simulink model "test_transform"  (R2018b)
settings: Solver=FixedStepAuto  StartTime=0  StopTime=5  FixedStep=Ts  RelTol=1e-3
values from neighbouring files (symbols this model uses):
  x_e = x_e_1    [AcDcInterlink.m]    (also in GridFollowingBuck.m; GridFormingBuck.m = [i_ld; i_lq; i_ld_i; i_lq_i; v_od; v_oq; v_od_i; v_oq_i; i_o)
undefined symbols (not defined in the file or in its folder): DeviceDiscreDamping, DevicePara, DevicePowerFlow, DeviceType, OtherInputs, PowerFlow, Sbase, Ts, Vbase, Wbase, Zbase
libraries: powerlib x11, SimplexPS x4
settings Model: Creator=yg934  LastModifiedBy=yg934

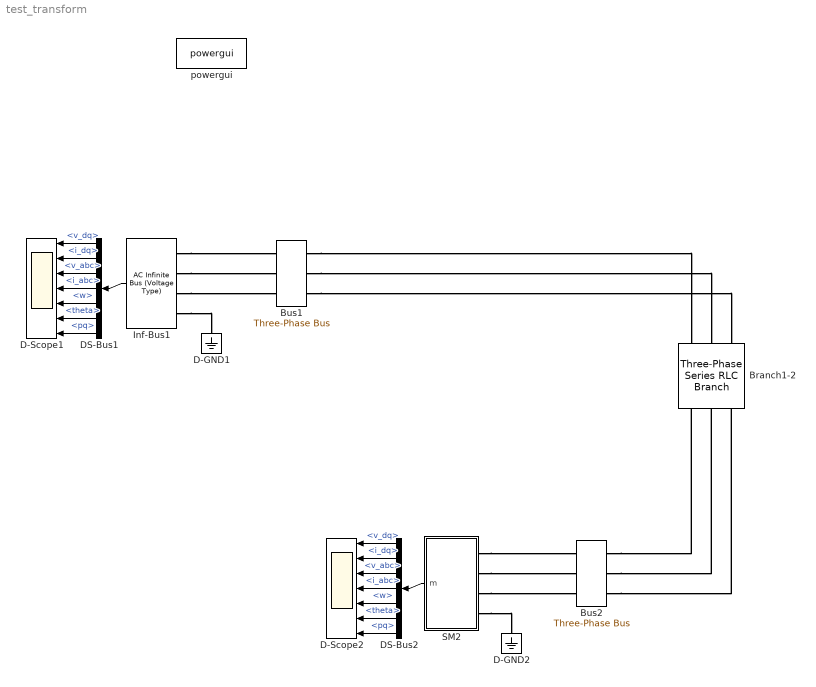
== system test_transform ==
  Branch1-2 : powerlib/Elements/Three-Phase Series RLC Branch  LConnTagsString=A|B|C  RConnTagsString=A|B|C  BranchType=L  Resistance=(0)*Zbase  Inductance=(0.65)*Zbase/Wbase  Capacitance=1e-6  Measurements=None
  Bus1 : SimplexPS/Three-Phase Bus  Vbase=1  Sbase=1
  Bus2 : SimplexPS/Three-Phase Bus  Vbase=1  Sbase=1
  D-GND1 : powerlib/Elements/Ground  LConnTagsString=a
  D-GND2 : powerlib/Elements/Ground  LConnTagsString=a
  D-Scope1 : Scope  NumInputPorts=7
  D-Scope2 : Scope  NumInputPorts=7
  DS-Bus1 : BusSelector  OutputSignals=v_dq,i_dq,v_abc,i_abc,w,theta,pq
  DS-Bus2 : BusSelector  OutputSignals=v_dq,i_dq,v_abc,i_abc,w,theta,pq
  Inf-Bus1 : SimplexPS/AC Infinite Bus (Voltage Type)  Ts=Ts  Sbase=Sbase  Vbase=Vbase  Wbase=Wbase  vd=PowerFlow{1}(3)  vq=0  theta0=PowerFlow{1}(4)  w=Wbase  R=1e-30
  SM2 : Subsystem  AncestorBlock=|  mask{Ts=Ts, Sbase=Sbase, Vbase=Vbase, Wbase=Wbase, DeviceType=DeviceType{2}, DevicePara=DevicePara{2}, PowerFlow=DevicePowerFlow{2}, x0=x_e{2}, OtherInputs=OtherInputs{2}, DiscreMethod=Hybrid Trapezoidal, EnableInsideModification=off, DiscreDampingFlag=on, DiscreDampingValue=DeviceDiscreDamping{2}, LinearizationTimes=1, DirectFeedthrough=off}
      | SimplexPS/Synchronous Machine
      | (dq-Frame System Object)
      mask prompts: Ts "Ts (s), samping period"; Sbase "Sbase (VA), power base"; Vbase "Vbase (V), voltage base"; Wbase "Wbase (rad/s), frequency base"; DeviceType "Device type"; DevicePara "Device parameters"; PowerFlow "Power flow paramters"; x0 "x0, initial states"; OtherInputs "Other inputs"; DiscreMethod "Discrerization method"; EnableInsideModification "Enable inside modification"; DiscreDampingFlag "Enable discretization damping"; DiscreDampingValue "Discretization damping value"; LinearizationTimes "Linearization times"; DirectFeedthrough "Direct feedthrough"
      mask init:
      | SimplexPS.Simulink.DeviceMaskInitialization(EnableInsideModification,DiscreDampingFlag);
      mask TypeOptions DiscreMethod: Forward Euler | Hybrid Trapezoidal | Virtual Damping
      mask TypeOptions LinearizationTimes: 1 | 2
  powergui : powerlib/powergui  Priority=1  SimulationMode=Discrete  SampleTime=Ts  frequency=60  Iterations=50  frequencyindice=0  Pbase=100e6  ErrMax=1e-4  UnitsV=kV  UnitsW=MW  buscounter=0  FunctionMessages=off  echomessages=off  EnableUseOfTLC=off  CurrentSourceSwitches=off  DisableSnubberDevices=off  DisableRonSwitches=off  DisableVfSwitches=off  DisplayEquations=off  SolverType=Tustin/Backward Euler (TBE)  Interpol=off  ExternalGateDelay=off  methode=off  Ts=100  x0status=blocks  SPID=off  SwTol=0  HookPort=off  RestoreLinks=warning  ResistiveCurrentMeasurement=off  Frange=[0:2:500]  Ylog=off  Xlog=on  ShowGrid=off  save=off  variable=ZData  structure=0  ZoomFFT=off  StartTime=0.0  cycles=1  DisplayStyle=1  fundamental=60  FreqAxis=off  MaxFrequency=1000  frequencyindicesteady=1  RmsSteady=1  display=off
  wires:
  Inf-Bus1/1 -> DS-Bus1/1
  DS-Bus1/1 -> D-Scope1/1  "<v_dq>"
  DS-Bus1/2 -> D-Scope1/2  "<i_dq>"
  DS-Bus1/3 -> D-Scope1/3  "<v_abc>"
  DS-Bus1/4 -> D-Scope1/4  "<i_abc>"
  DS-Bus1/5 -> D-Scope1/5  "<w>"
  DS-Bus1/6 -> D-Scope1/6  "<theta>"
  DS-Bus1/7 -> D-Scope1/7  "<pq>"
  SM2/1(m) -> DS-Bus2/1
  DS-Bus2/1 -> D-Scope2/1  "<v_dq>"
  DS-Bus2/2 -> D-Scope2/2  "<i_dq>"
  DS-Bus2/3 -> D-Scope2/3  "<v_abc>"
  DS-Bus2/4 -> D-Scope2/4  "<i_abc>"
  DS-Bus2/5 -> D-Scope2/5  "<w>"
  DS-Bus2/6 -> D-Scope2/6  "<theta>"
  DS-Bus2/7 -> D-Scope2/7  "<pq>"
  connections:
  Inf-Bus1/LConn4 -- D-GND1/LConn1
  SM2/LConn4 -- D-GND2/LConn1
  Bus2/RConn1 -- Branch1-2/RConn1
  Bus2/RConn2 -- Branch1-2/RConn2
  Bus2/RConn3 -- Branch1-2/RConn3
  Bus1/RConn1 -- Branch1-2/LConn1
  Bus1/RConn2 -- Branch1-2/LConn2
  Bus1/RConn3 -- Branch1-2/LConn3
  Inf-Bus1/LConn1 -- Bus1/LConn1
  Inf-Bus1/LConn2 -- Bus1/LConn2
  Inf-Bus1/LConn3 -- Bus1/LConn3
  SM2/LConn1 -- Bus2/LConn1
  SM2/LConn2 -- Bus2/LConn2
  SM2/LConn3 -- Bus2/LConn3

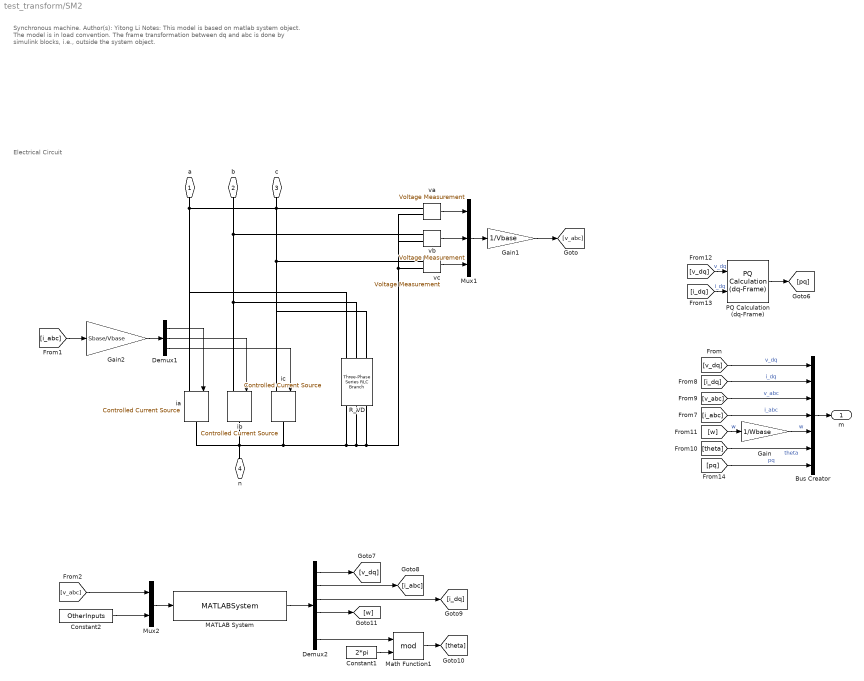
== system test_transform/SM2 ==
  note: Electrical Circuit
  note: Synchronous machine.
      |
      | Author(s): Yitong Li
      |
      | Notes:
      |
      | This model is based on matlab system object.
      |
      | The model is in load convention.
      |
      | The frame transformation between dq and abc is done by simulink blocks, i.e., outside the system object.
  Bus Creator : BusCreator  Inputs=7
  Constant1 : Constant  Value=2*pi
  Constant2 : Constant  Value=OtherInputs
  Demux1 : Demux  Outputs=3
  Demux2 : Demux  Outputs=[2,3,2,1,1,1]
  Gain : Gain  Gain=1/Wbase
  Gain1 : Gain  Gain=1/Vbase
  Gain2 : Gain  Gain=Sbase/Vbase
  MATLAB System : MATLABSystem  System=SimplexPS.Class.SynchronousMachineTransform  Ts=Ts  Para=DevicePara  DeviceType=DeviceType  PowerFlow=PowerFlow  x0=x0  DiscreMethod=DiscreMethod  LinearizationTimes=LinearizationTimes  DirectFeedthrough=DirectFeedthrough  VirtualResistor=DiscreDampingFlag  EquiInitial=true  ElecPortIOs=[ 1, 2 ]  SimulateUsing=Code generation
      mask Type: SimplexPS.Class.SynchronousMachineTransform
      mask Display:
      | disp('SynchronousMachineTransform');
      | port_label('input',1,'u');
      | port_label('output',1,'y');
  Math Function1 : Math  Operator=mod  SaturateOnIntegerOverflow=on
  Mux1 : Mux  Inputs=3
  Mux2 : Mux  Inputs=[3,2]
  PQ Calculation (dq-Frame) : SimplexPS/PQ Calculation (dq-Frame)  SystemSampleTime=-1
  R_VD : powerlib/Elements/Three-Phase Series RLC Branch  LConnTagsString=A|B|C  RConnTagsString=A|B|C  BranchType=R  Resistance=DiscreDampingValue*Vbase^2/Sbase  Inductance=1e-3  Capacitance=1e-6  Measurements=None
  ia : powerlib/Electrical Sources/Controlled Current Source  Initialize=on  Source_Type=AC  Amplitude=0  Phase=0  Frequency=0  Measurements=None
  ib : powerlib/Electrical Sources/Controlled Current Source  Initialize=on  Source_Type=AC  Amplitude=0  Phase=0  Frequency=0  Measurements=None
  ic : powerlib/Electrical Sources/Controlled Current Source  Initialize=on  Source_Type=AC  Amplitude=0  Phase=0  Frequency=0  Measurements=None
  va : powerlib/Measurements/Voltage Measurement  PhasorSimulation=off  OutputType=Complex  PSBequivalent=0
  vb : powerlib/Measurements/Voltage Measurement  PhasorSimulation=off  OutputType=Complex  PSBequivalent=0
  vc : powerlib/Measurements/Voltage Measurement  PhasorSimulation=off  OutputType=Complex  PSBequivalent=0
  a : PMIOPort  Side=Left
  b : PMIOPort  Port=2  Side=Left
  c : PMIOPort  Port=3  Side=Left
  n : PMIOPort  Port=4  Side=Left
  m : Outport
  wires:
  Gain2/1 -> Demux1/1
  Gain1/1 -> [v_abc]
  [pq] -> Bus Creator/7  "pq"
  PQ Calculation (dq-Frame)/1 -> [pq]
  [i_dq] -> PQ Calculation (dq-Frame)/2  "i_dq"
  [v_dq] -> PQ Calculation (dq-Frame)/1  "v_dq"
  [i_abc] -> Gain2/1
  Mux1/1 -> Gain1/1
  Gain/1 -> Bus Creator/5  "w"
  Bus Creator/1 -> m/1
  [theta] -> Bus Creator/6  "theta"
  [w] -> Gain/1  "w"
  [i_abc] -> Bus Creator/4  "i_abc"
  [v_abc] -> Bus Creator/3  "v_abc"
  [i_dq] -> Bus Creator/2  "i_dq"
  [v_dq] -> Bus Creator/1  "v_dq"
  Demux1/3 -> ic/1
  vc/1 -> Mux1/3
  Mux2/1 -> MATLAB System/1
  [v_abc] -> Mux2/1
  vb/1 -> Mux1/2
  va/1 -> Mux1/1
  Demux1/2 -> ib/1
  Demux1/1 -> ia/1
  Constant2/1 -> Mux2/2
  Demux2/1 -> [v_dq]
  Demux2/2 -> [i_abc]
  Demux2/3 -> [i_dq]
  Math Function1/1 -> [theta]
  Constant1/1 -> Math Function1/2
  Demux2/6 -> Math Function1/1
  Demux2/4 -> [w]
  MATLAB System/1 -> Demux2/1
  connections:
  c/RConn1 -- ic/LConn1 -- R_VD/LConn3 -- vc/LConn1
  vb/LConn1 -- ib/LConn1 -- R_VD/LConn2 -- b/RConn1
  va/LConn1 -- ia/LConn1 -- R_VD/LConn1 -- a/RConn1
  ic/RConn1 -- n/RConn1 -- ib/RConn1 -- ia/RConn1 -- R_VD/RConn1 -- R_VD/RConn2 -- R_VD/RConn3 -- vc/LConn2 -- va/LConn2 -- vb/LConn2
